simulink model "pacemaker_model"  (R2023a)
settings: Solver=FixedStepAuto  StartTime=0.0  StopTime=10.0  FixedStep=1e-3  RelTol=1e-3  EnableMultiTasking=on
settings Model: ExtModeTrigDuration=5  Creator=emcan  LastModifiedBy=emcan
settings OptimizationCC: EnhancedBackFolding=on  PassReuseOutputArgsAs=Individual arguments  ZeroExternalMemoryAtStartup=off  ZeroInternalMemoryAtStartup=off  MaxStackSize=64  OptimizeBlockOrder=speed  DifferentSizesBufferReuse=on  OptimizationCustomize=off  EfficientTunableParamExpr=on
settings DebuggingCC: ParameterTunabilityLossMsg=error
settings HardwareCC: ProdBitPerPointer=32  ProdBitPerSizeT=32  ProdBitPerPtrDiffT=32  ProdLargestAtomicInteger=Long  ProdLargestAtomicFloat=Double  ProdWordSize=32  ProdHWDeviceType=ARM Compatible->ARM Cortex
settings SFSimCC: MATLABDynamicMemAlloc=off
settings RTWCC: Description=Embedded Coder  SystemTargetFile=ert.tlc  HardwareBoard=NXP FRDM-K64F  TLCOptions="-aInlineSetEventsForThisBaseRateFcn=TLC_FALSE -aSuppressMultiTaskScheduler=TLC_FALSE  -aRateBasedStepFcn=0"  TemplateMakefile=ert_default_tmf  Toolchain=GNU Tools for ARM Embedded Processors
settings CodeAppCC: ForceParamTrailComments=on  IgnoreCustomStorageClasses=off  OperatorAnnotations=on  SimulinkDataObjDesc=on  SFDataObjDesc=on  InsertBlockDesc=on
settings ERTTargetCC: ExtModeTransport=4  ExtModeMexFile=sendToCommService

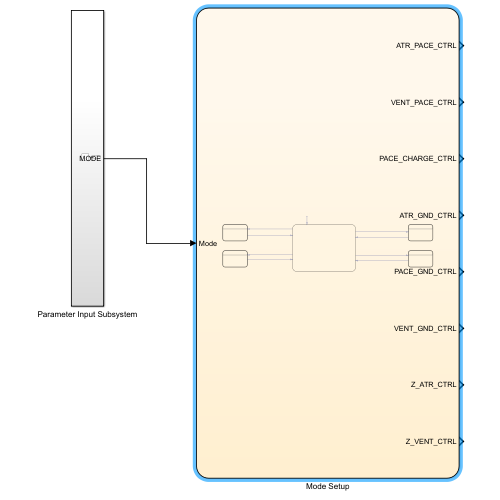
[thumbnail: Simulink's stored preview of the top-level diagram]
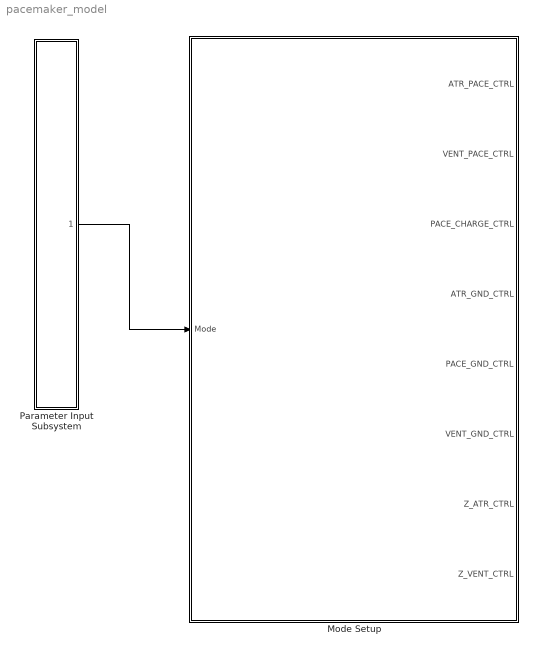
== system pacemaker_model ==
  Mode Setup : Stateflow chart  TreatAsAtomicUnit=on
  Parameter Input Subsystem : Subsystem
  wires:
  Parameter Input Subsystem/1(MODE) -> Mode Setup/1(Mode)

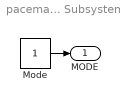
== system pacemaker_model/Parameter Input Subsystem ==
  Mode : Constant  OutDataTypeStr=uint8
  MODE : Outport
  wires:
  Mode/1 -> MODE/1

== stateflow chart pacemaker_model/Mode Setup ==
  state AOO
    state Charging_C22_and_Discharging_Blocking_Cap
      entry:
      %% Charging C22
      ATR_PACE_CTRL = false;
      VENT_PACE_CTRL = false;
      %PACING_REF_PWM = ????
      PACE_CHARGE_CTRL = true;
      %% Discharging Blocking Capacitor
      PACE_GND_CTRL = true;
      %VENT_PACE_CTRL = false;
      Z_ATR_CTRL = false;
      Z_VENT_CTRL = false;
      %ATR_PACE_CTRL = false;
      ATR_GND_CTRL = true;
      VENT_GND_CTRL = false;
    state Discharging_C22_into_AV
      entry:
      %% Discharge
      PACE_CHARGE_CTRL = false;
      %PACE_GND_CTRL = true;
      ATR_PACE_CTRL = true;
      ATR_GND_CTRL = false;
      %Z_ATR_CTRL = false;
      %Z_VENT_CTRL = false;
      %VENT_GND_CTRL = false;
      %VENT_PACE_CTRL = false;
    (default) -> Charging_C22_and_Discharging_Blocking_Cap
    Charging_C22_and_Discharging_Blocking_Cap -> Discharging_C22_into_AV
    Discharging_C22_into_AV -> Charging_C22_and_Discharging_Blocking_Cap
  state Mode
    %% 0: AOO
    %% 1: VOO
    %% 2: AAI
    %% 3: VVI
  state VOO
  state AAI
  state VVI
  (default) -> Mode
  Mode -> AOO [order 1] : [Mode == 0]
  Mode -> VOO [order 2] : [Mode == 1]
  AOO -> Mode : [Mode ~= 0]
  VOO -> Mode : [Mode ~= 1]
  Mode -> AAI [order 3] : [Mode == 2]
  Mode -> VVI [order 4] : [Mode == 3]
  AAI -> Mode : [Mode ~= 2]
  VVI -> Mode : [Mode ~= 3]
  data: Mode input; ATR_PACE_CTRL output; VENT_PACE_CTRL output; PACE_CHARGE_CTRL output; ATR_GND_CTRL output; PACE_GND_CTRL output; VENT_GND_CTRL output; Z_ATR_CTRL output; Z_VENT_CTRL output
